simulink model "CL_pitch_reference_generator_discrete"  (R2016b)
settings: Solver=FixedStepAuto  StartTime=0.0  StopTime=10.0  FixedStep=1/512  RelTol=1e-3
undefined symbols (not defined in the file or in its folder): DiscIntNeverNeededParam
settings Model: Creator=kmkajak  LastModifiedBy=Karl

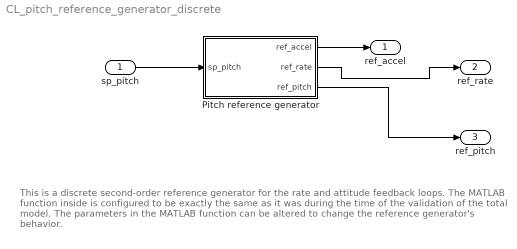
== system CL_pitch_reference_generator_discrete ==
  note: This is a discrete second-order reference generator for the rate and attitude feedback loops. The MATLAB function inside is configured to
      | be exactly the same as it was during the time of the validation of the total model. The parameters in the MATLAB function can be altered to
      | change the reference generator's behavior.
  sp_pitch : Inport
  Pitch reference generator : Subsystem
  ref_accel : Outport
  ref_rate : Outport  Port=2
  ref_pitch : Outport  Port=3
  wires:
  sp_pitch/1 -> Pitch reference generator/1(sp_pitch)
  Pitch reference generator/1(ref_accel) -> ref_accel/1
  Pitch reference generator/2(ref_rate) -> ref_rate/1
  Pitch reference generator/3(ref_pitch) -> ref_pitch/1

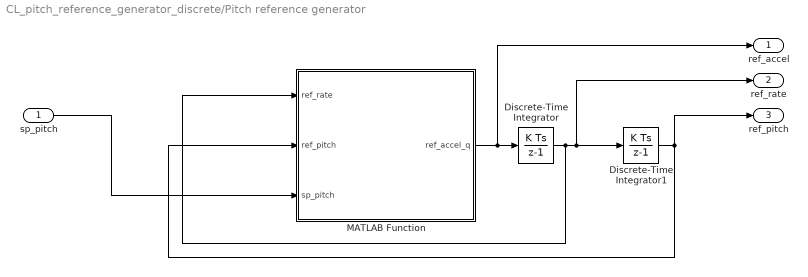
== system CL_pitch_reference_generator_discrete/Pitch reference generator ==
  sp_pitch : Inport
  Discrete-Time Integrator : DiscreteIntegrator  gainval=1  InitialConditionSetting=State (most efficient)  SampleTime=-1  ICPrevOutput=DiscIntNeverNeededParam  ICPrevScaledInput=DiscIntNeverNeededParam
  Discrete-Time Integrator1 : DiscreteIntegrator  gainval=1  InitialConditionSetting=State (most efficient)  SampleTime=-1  ICPrevOutput=DiscIntNeverNeededParam  ICPrevScaledInput=DiscIntNeverNeededParam
  MATLAB Function : MATLAB Function  TreatAsAtomicUnit=on  SystemSampleTime=1/512
  ref_accel : Outport
  ref_rate : Outport  Port=2
  ref_pitch : Outport  Port=3
  wires:
  MATLAB Function/1(ref_accel_q) -> Discrete-Time Integrator/1, ref_accel/1
  Discrete-Time Integrator/1 -> Discrete-Time Integrator1/1, ref_rate/1, MATLAB Function/1(ref_rate)
  Discrete-Time Integrator1/1 -> ref_pitch/1, MATLAB Function/2(ref_pitch)
  sp_pitch/1 -> MATLAB Function/3(sp_pitch)

== matlab function CL_pitch_reference_generator_discrete/Pitch reference generator/MATLAB Function ==
  data: ref_rate input; ref_accel_q output; ref_pitch input; sp_pitch input
function ref_accel_q = fcn(ref_rate, ref_pitch, sp_pitch)
ref_err_theta = ref_pitch - sp_pitch;

ref_zeta_q = 0.85;
ref_omega_q = 800/180*pi; %deg/s
ref_max_q = 400/180*pi; %deg/s
ref_max_accel_q = 8000/180*pi; % rad



ref_accel_q = -2*ref_zeta_q*ref_omega_q*ref_rate - ref_omega_q^2*ref_err_theta;


% saturate rate
if ref_rate > ref_max_q
    ref_rate = ref_max_q;
    if ref_accel_q > 0
        ref_accel_q = 0;
    end
end
if ref_rate < -ref_max_q
    ref_rate = -ref_max_q;
    if ref_accel_q < 0
        ref_accel_q = 0;
    end
end

% saturate acceleration
if ref_accel_q > ref_max_accel_q
    ref_accel_q = ref_max_accel_q;
end
if ref_accel_q < -ref_max_accel_q
    ref_accel_q = -ref_max_accel_q;
end
